simulink model "F1_Telemetry_UDP_Fix"  (R2025a)
settings: Solver=FixedStepAuto  StartTime=0.0  StopTime=inf  FixedStep=0.05  RelTol=1e-3
settings Model: Creator=sunda  LastModifiedBy=sunda

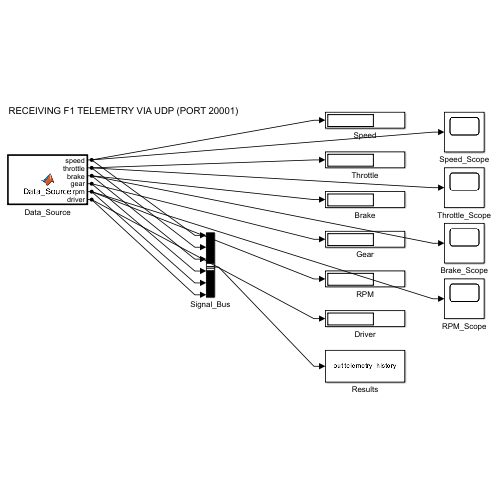
[thumbnail: Simulink's stored preview of the top-level diagram]
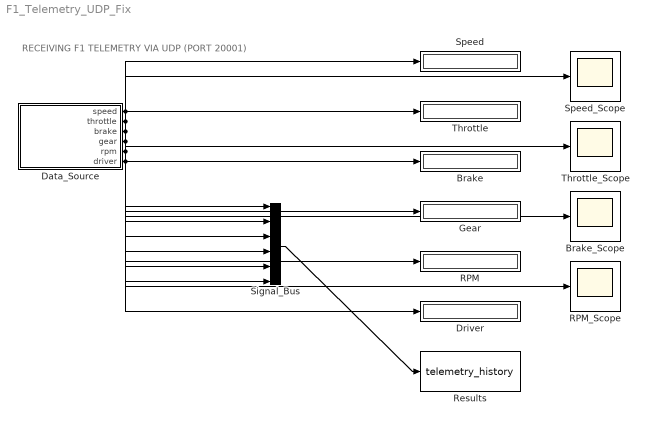
== system F1_Telemetry_UDP_Fix ==
  note: RECEIVING F1 TELEMETRY VIA UDP (PORT 20001)
  Brake : Display
  Brake_Scope : Scope
  Data_Source : MATLAB Function  TreatAsAtomicUnit=on
  Driver : Display
  Gear : Display
  RPM : Display
  RPM_Scope : Scope
  Results : ToWorkspace  VariableName=telemetry_history  SaveFormat=Timeseries  SampleTime=-1
  Signal_Bus : BusCreator  Inputs=6
  Speed : Display
  Speed_Scope : Scope
  Throttle : Display
  Throttle_Scope : Scope
  wires:
  Data_Source/1(speed) -> Speed/1, Speed_Scope/1, Signal_Bus/1
  Data_Source/2(throttle) -> Throttle/1, Throttle_Scope/1, Signal_Bus/2
  Data_Source/3(brake) -> Brake/1, Brake_Scope/1, Signal_Bus/3
  Data_Source/4(gear) -> Gear/1, Signal_Bus/4
  Data_Source/5(rpm) -> RPM/1, RPM_Scope/1, Signal_Bus/5
  Data_Source/6(driver) -> Driver/1, Signal_Bus/6
  Signal_Bus/1 -> Results/1

== matlab function F1_Telemetry_UDP_Fix/Data_Source ==
  data: speed output; throttle output; brake output; gear output; rpm output; driver output
function [speed, throttle, brake, gear, rpm, driver] = Data_Source()
    % Access global telemetry data that is updated by the UDP receiver
    global telemetry_data;
    
    % Extract values from telemetry data struct
    speed = double(telemetry_data.speed);
    throttle = double(telemetry_data.throttle);
    brake = double(telemetry_data.brake);
    gear = double(telemetry_data.gear);
    rpm = double(telemetry_data.rpm);
    driver = double(telemetry_data.driver);
end
